simulink model "test"  (Simulink 3.00)
settings: Solver=FixedStepDiscrete  StartTime=0.0  StopTime=60  FixedStep=.0005  RelTol=1e-3

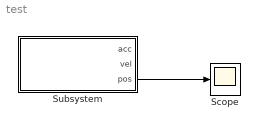
== system test ==
  Scope : Scope
      settings: TimeRange=60  YMin=2.5  YMax=30  SaveToWorkspace=off  SaveName=ScopeData
  Subsystem : Subsystem
      settings: OpenFcn=r3g_main
      mask Type: Ref3
      mask Display: disp('Ref3');
  wires:
  Subsystem/3(pos) -> Scope/1

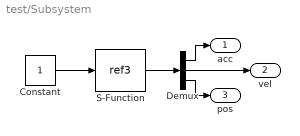
== system test/Subsystem ==
  Constant : Constant  Value=1
  Demux : Demux  Outputs=3
  S-Function : S-Function  FunctionName=ref3  Parameters=ref_part  PortCounts=[]  SFunctionModules=''
      settings: OpenFcn=global ref_part; r3g_main
  acc : Outport  Port=1
  vel : Outport  Port=2
  pos : Outport  Port=3
  wires:
  Constant/1 -> S-Function/1
  S-Function/1 -> Demux/1
  Demux/1 -> acc/1
  Demux/2 -> vel/1
  Demux/3 -> pos/1
